simulink model "DerivedTransferFunctions"  (R2018b)
settings: Solver=VariableStepAuto  StartTime=0.0  StopTime=10  RelTol=1e-3
InitFcn:
  | SimFramework('model_parameters.json');
model workspace (MAT data in the model file):
  D = 0.5
  Fsin = 1
  Fstep = 10
  FstepOffTime = 5
  FstepOnTime = 1
  K = 500
  K1 = 5
  L = 0.0005
  R = 75
  StopTime = 6
  Vb = 0.1
  Vsin = 1
  Vstep = 1
  VstepOffTime = 100
  VstepOnTime = 1
  couple = 1
  freq = 1000
  m = 0.004
  name = 'DerivedTransferFunctions'
  step = 1
settings Model: Creator=franboonham  LastModifiedBy=franboonham
settings DataIOCC: ReturnWorkspaceOutputs=on

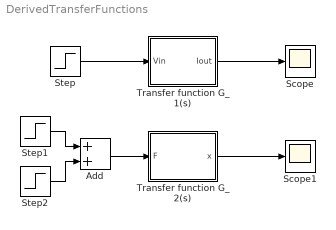
== system DerivedTransferFunctions ==
  Add : Sum
  Scope : Scope
  Scope1 : Scope
  Step : Step  SampleTime=0
  Step1 : Step  After=10  SampleTime=0
  Step2 : Step  Time=5  After=-10  SampleTime=0
  Transfer function G_1(s) : Subsystem
  Transfer function G_2(s) : Subsystem
  wires:
  Step/1 -> Transfer function G_1(s)/1(Vin)
  Transfer function G_1(s)/1(Iout) -> Scope/1
  Transfer function G_2(s)/1(x) -> Scope1/1
  Step1/1 -> Add/1
  Step2/1 -> Add/2
  Add/1 -> Transfer function G_2(s)/1(F)

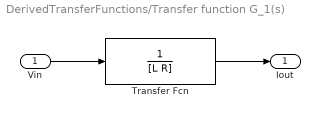
== system DerivedTransferFunctions/Transfer function G_1(s) ==
  Vin : Inport
  Transfer Fcn : TransferFcn  Denominator=[L R]
  Iout : Outport
  wires:
  Vin/1 -> Transfer Fcn/1
  Transfer Fcn/1 -> Iout/1

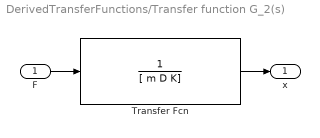
== system DerivedTransferFunctions/Transfer function G_2(s) ==
  F : Inport
  Transfer Fcn : TransferFcn  Denominator=[ m D K]
  x : Outport
  wires:
  F/1 -> Transfer Fcn/1
  Transfer Fcn/1 -> x/1
